simulink model "second_order_follow"  (R2023b)
settings: Solver=VariableStepAuto  StartTime=0.0  StopTime=30  RelTol=1e-3
libraries: simulink x2
settings Model: Creator=Maxwe  LastModifiedBy=Maxwe

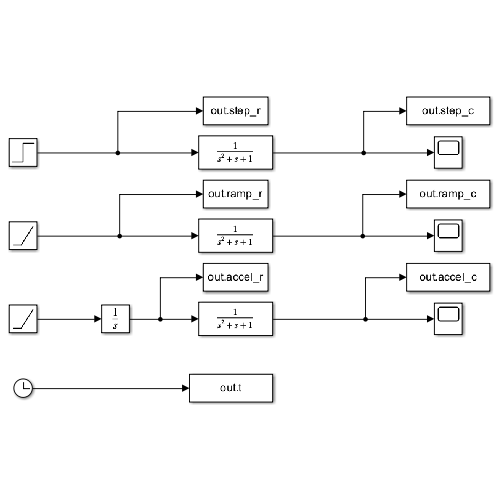
[thumbnail: Simulink's stored preview of the top-level diagram]
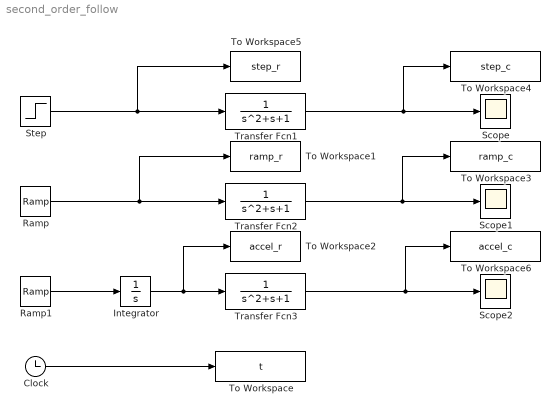
== system second_order_follow ==
  Clock : Clock
  Integrator : Integrator
  Ramp : simulink/Sources/Ramp  slope=1  start=0  InitialOutput=0
  Ramp1 : simulink/Sources/Ramp  slope=1  start=0  InitialOutput=0
  Scope : Scope
  Scope1 : Scope
  Scope2 : Scope
  Step : Step  SampleTime=0
  To Workspace : ToWorkspace  VariableName=t  SampleTime=-1
      settings: Save2DSignal=2-D array (concatenate along first dimension)
  To Workspace1 : ToWorkspace  VariableName=ramp_r  SampleTime=-1
      settings: Save2DSignal=2-D array (concatenate along first dimension)
  To Workspace2 : ToWorkspace  VariableName=accel_r  SampleTime=-1
      settings: Save2DSignal=2-D array (concatenate along first dimension)
  To Workspace3 : ToWorkspace  VariableName=ramp_c  SampleTime=-1
      settings: Save2DSignal=2-D array (concatenate along first dimension)
  To Workspace4 : ToWorkspace  VariableName=step_c  SampleTime=-1
      settings: Save2DSignal=2-D array (concatenate along first dimension)
  To Workspace5 : ToWorkspace  VariableName=step_r  SampleTime=-1
      settings: Save2DSignal=2-D array (concatenate along first dimension)
  To Workspace6 : ToWorkspace  VariableName=accel_c  SampleTime=-1
      settings: Save2DSignal=2-D array (concatenate along first dimension)
  Transfer Fcn1 : TransferFcn  Numerator=[0 1]  Denominator=[1 1 1]
  Transfer Fcn2 : TransferFcn  Numerator=[0 1]  Denominator=[1 1 1]
  Transfer Fcn3 : TransferFcn  Numerator=[0 1]  Denominator=[1 1 1]
  wires:
  Step/1 -> Transfer Fcn1/1, To Workspace5/1
  Clock/1 -> To Workspace/1
  Ramp/1 -> To Workspace1/1, Transfer Fcn2/1
  Ramp1/1 -> Integrator/1
  Integrator/1 -> To Workspace2/1, Transfer Fcn3/1
  Transfer Fcn3/1 -> Scope2/1, To Workspace6/1
  Transfer Fcn2/1 -> Scope1/1, To Workspace3/1
  Transfer Fcn1/1 -> To Workspace4/1, Scope/1
